simulink library "AtomicLibrary"
PostLoadFcn:
  | PacketBusGenerator; RailCabBusGenerator
(part 3 of 8)

== system AtomicLibrary/TestStartStopMaster/Link Layer startStop_Master ==
  port_in : Inport  Tag=id=_rqhdoPdmEeGH_6eRdlYQdA  Port=1  PortDimensions=-1  DataType=auto  OutDataType=fixdt(1, 16)  OutScaling=2^0  UseBusObject=on  OutDataTypeStr=Inherit: auto
      settings: BusObject=PacketBus
  net_address : Inport  Tag=id=_rqrOoPdmEeGH_6eRdlYQdA  Port=2  PortDimensions=-1  DataType=uint8  OutDataType=fixdt(1, 16)  OutScaling=2^0  OutDataTypeStr=uint8
  receiver_net_address : Inport  Tag=id=_rqr1sPdmEeGH_6eRdlYQdA  Port=3  PortDimensions=-1  DataType=uint8  OutDataType=fixdt(1, 16)  OutScaling=2^0  OutDataTypeStr=uint8
  read_event_queue_in : Inport  Tag=id=_rqiEsPdmEeGH_6eRdlYQdA  Port=4  PortDimensions=-1  DataType=auto  OutDataType=fixdt(1, 16)  OutScaling=2^0  OutDataTypeStr=Inherit: auto
  read_event_param_queue_in : Inport  Tag=id=_rqlvEPdmEeGH_6eRdlYQdA  Port=5  PortDimensions=-1  DataType=auto  OutDataType=fixdt(1, 16)  OutScaling=2^0  OutDataTypeStr=Inherit: auto
  read_event_queue_out : Inport  Tag=id=_rqnkQPdmEeGH_6eRdlYQdA  Port=6  PortDimensions=-1  DataType=auto  OutDataType=fixdt(1, 16)  OutScaling=2^0  OutDataTypeStr=Inherit: auto
  read_event_param_queue_out : Inport  Tag=id=_rqoyYPdmEeGH_6eRdlYQdA  Port=7  PortDimensions=-1  DataType=auto  OutDataType=fixdt(1, 16)  OutScaling=2^0  OutDataTypeStr=Inherit: auto
  port_out : Outport  Tag=id=_rqgPgPdmEeGH_6eRdlYQdA  Port=1  PortDimensions=-1  DataType=auto  OutDataType=fixdt(1, 16)  OutScaling=2^0  UseBusObject=on  OutDataTypeStr=Inherit: auto
      settings: BusObject=PacketBus
  write_event_queue_in : Outport  Tag=id=_rqjS0PdmEeGH_6eRdlYQdA  Port=2  PortDimensions=-1  DataType=auto  OutDataType=fixdt(1, 16)  OutScaling=2^0  OutDataTypeStr=Inherit: auto
  write_event_param_queue_in : Outport  Tag=id=_rqkg8PdmEeGH_6eRdlYQdA  Port=3  PortDimensions=-1  DataType=auto  OutDataType=fixdt(1, 16)  OutScaling=2^0  OutDataTypeStr=Inherit: auto
  write_event_queue_out : Outport  Tag=id=_rqpZcPdmEeGH_6eRdlYQdA  Port=4  PortDimensions=-1  DataType=auto  OutDataType=fixdt(1, 16)  OutScaling=2^0  OutDataTypeStr=Inherit: auto
  write_event_param_queue_out : Outport  Tag=id=_rqqAgPdmEeGH_6eRdlYQdA  Port=5  PortDimensions=-1  DataType=auto  OutDataType=fixdt(1, 16)  OutScaling=2^0  OutDataTypeStr=Inherit: auto
  DataLinkLayer : Subsystem  Tag=id=_rqtq4PdmEeGH_6eRdlYQdA
  Bus Selector : BusSelector  OutputSignals=from,to,msg,param,pkgid,time  Tag=id=_rqtD0PdmEeGH_6eRdlYQdA
  Unit Delay1 : UnitDelay  Tag=id=_rqtD0fdmEeGH_6eRdlYQdA  SampleTime=-1
  Unit Delay2 : UnitDelay  Tag=id=_rqtD0vdmEeGH_6eRdlYQdA  SampleTime=-1
  Unit Delay3 : UnitDelay  Tag=id=_rqtq4fdmEeGH_6eRdlYQdA  SampleTime=-1
  Bus Creator : BusCreator  Inputs=6  UseBusObject=on  Tag=id=_rquR8PdmEeGH_6eRdlYQdA
      settings: BusObject=PacketBus
  Unit Delay4 : UnitDelay  Tag=id=_rquR8fdmEeGH_6eRdlYQdA  SampleTime=-1
  Terminator : Terminator
      settings: Tag=id=_rquR8vdmEeGH_6eRdlYQdA
  Receive Packet : Stateflow chart  Tag=id=_rqu5APdmEeGH_6eRdlYQdA
  Send Packet : Stateflow chart  Tag=id=_rqu5AfdmEeGH_6eRdlYQdA
  wires:
  DataLinkLayer/3(snd_msg_out) -> Bus Creator/3
  DataLinkLayer/8(recv_msg_out) -> Receive Packet/2(packetMsg)
  Send Packet/3(eventQueue) -> Unit Delay1/1
  DataLinkLayer/7(recv_from_out) -> Receive Packet/1(packetFrom)
  Bus Selector/3 -> DataLinkLayer/3(recv_msg_in)
  read_event_param_queue_in/1 -> Receive Packet/5(eventParamQueueIn)
  Receive Packet/3(bufferOverflow) -> Terminator/1
  receiver_net_address/1 -> DataLinkLayer/8(snd_to_in)
  Receive Packet/2(eventParamQueue) -> Unit Delay4/1
  read_event_queue_out/1 -> Send Packet/2(eventQueueIn)
  DataLinkLayer/9(recv_param_out) -> Receive Packet/3(packetParam)
  Send Packet/2(packetParam) -> DataLinkLayer/10(snd_param_in)
  Bus Selector/2 -> DataLinkLayer/2(recv_to_in)
  port_in/1 -> Bus Selector/1
  read_event_param_queue_out/1 -> Send Packet/3(eventParamQueueIn)
  Send Packet/4(eventParamQueue) -> Unit Delay2/1
  Bus Selector/5 -> DataLinkLayer/5(recv_pkgid_in)
  Unit Delay4/1 -> write_event_param_queue_in/1
  read_event_queue_in/1 -> Receive Packet/4(eventQueueIn)
  Bus Selector/4 -> DataLinkLayer/4(recv_param_in)
  DataLinkLayer/2(snd_to_out) -> Bus Creator/2
  Bus Selector/6 -> DataLinkLayer/6(recv_time_in), Send Packet/1(busSizeSignal)
  Receive Packet/1(eventQueue) -> Unit Delay3/1
  DataLinkLayer/6(snd_time_out) -> Bus Creator/6
  Unit Delay1/1 -> write_event_queue_out/1
  DataLinkLayer/1(snd_from_out) -> Bus Creator/1
  DataLinkLayer/5(snd_pkgid_out) -> Bus Creator/5
  net_address/1 -> DataLinkLayer/7(snd_from_in)
  Send Packet/1(packetMsg) -> DataLinkLayer/9(snd_msg_in)
  Bus Creator/1 -> port_out/1  "Outport37"
  Unit Delay3/1 -> write_event_queue_in/1
  Bus Selector/1 -> DataLinkLayer/1(recv_from_in)
  Unit Delay2/1 -> write_event_param_queue_out/1
  DataLinkLayer/4(snd_param_out) -> Bus Creator/4

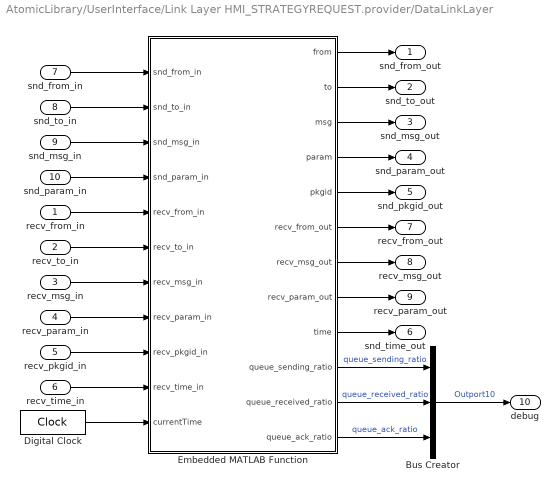
== system AtomicLibrary/UserInterface/Link Layer HMI_STRATEGYREQUEST.provider/DataLinkLayer ==
  recv_from_in : Inport  Tag=id=_r1VmgPdmEeGH_6eRdlYQdA  Port=1  PortDimensions=-1  DataType=uint8  OutDataType=fixdt(1, 16)  OutScaling=2^0  OutDataTypeStr=uint8
  recv_to_in : Inport  Tag=id=_r1XbsPdmEeGH_6eRdlYQdA  Port=2  PortDimensions=-1  DataType=uint8  OutDataType=fixdt(1, 16)  OutScaling=2^0  OutDataTypeStr=uint8
  recv_msg_in : Inport  Tag=id=_r1Yp0PdmEeGH_6eRdlYQdA  Port=3  PortDimensions=-1  DataType=uint16  OutDataType=fixdt(1, 16)  OutScaling=2^0  OutDataTypeStr=uint16
  recv_param_in : Inport  Tag=id=_r1afAPdmEeGH_6eRdlYQdA  Port=4  PortDimensions=-1  DataType=double  OutDataType=fixdt(1, 16)  OutScaling=2^0  OutDataTypeStr=double
  recv_pkgid_in : Inport  Tag=id=_r1cUMPdmEeGH_6eRdlYQdA  Port=5  PortDimensions=-1  DataType=uint32  OutDataType=fixdt(1, 16)  OutScaling=2^0  OutDataTypeStr=uint32
  recv_time_in : Inport  Tag=id=_r1eJYPdmEeGH_6eRdlYQdA  Port=6  PortDimensions=-1  DataType=double  OutDataType=fixdt(1, 16)  OutScaling=2^0  OutDataTypeStr=double
  snd_from_in : Inport  Tag=id=_r1f-kPdmEeGH_6eRdlYQdA  Port=7  PortDimensions=-1  DataType=uint8  OutDataType=fixdt(1, 16)  OutScaling=2^0  OutDataTypeStr=uint8
  snd_to_in : Inport  Tag=id=_r1hzwPdmEeGH_6eRdlYQdA  Port=8  PortDimensions=-1  DataType=uint8  OutDataType=fixdt(1, 16)  OutScaling=2^0  OutDataTypeStr=uint8
  snd_msg_in : Inport  Tag=id=_r1jo8PdmEeGH_6eRdlYQdA  Port=9  PortDimensions=-1  DataType=uint16  OutDataType=fixdt(1, 16)  OutScaling=2^0  OutDataTypeStr=uint16
  snd_param_in : Inport  Tag=id=_r1leIPdmEeGH_6eRdlYQdA  Port=10  PortDimensions=-1  DataType=double  OutDataType=fixdt(1, 16)  OutScaling=2^0  OutDataTypeStr=double
  snd_from_out : Outport  Tag=id=_r1LOcPdmEeGH_6eRdlYQdA  Port=1  PortDimensions=-1  DataType=uint8  OutDataType=fixdt(1, 16)  OutScaling=2^0  OutDataTypeStr=uint8
  snd_to_out : Outport  Tag=id=_r1L1gPdmEeGH_6eRdlYQdA  Port=2  PortDimensions=-1  DataType=uint8  OutDataType=fixdt(1, 16)  OutScaling=2^0  OutDataTypeStr=uint8
  snd_msg_out : Outport  Tag=id=_r1NDoPdmEeGH_6eRdlYQdA  Port=3  PortDimensions=-1  DataType=uint16  OutDataType=fixdt(1, 16)  OutScaling=2^0  OutDataTypeStr=uint16
  snd_param_out : Outport  Tag=id=_r1ORwPdmEeGH_6eRdlYQdA  Port=4  PortDimensions=-1  DataType=double  OutDataType=fixdt(1, 16)  OutScaling=2^0  OutDataTypeStr=double
  snd_pkgid_out : Outport  Tag=id=_r1Pf4PdmEeGH_6eRdlYQdA  Port=5  PortDimensions=-1  DataType=uint32  OutDataType=fixdt(1, 16)  OutScaling=2^0  OutDataTypeStr=uint32
  snd_time_out : Outport  Tag=id=_r1QG8PdmEeGH_6eRdlYQdA  Port=6  PortDimensions=-1  DataType=double  OutDataType=fixdt(1, 16)  OutScaling=2^0  OutDataTypeStr=double
  recv_from_out : Outport  Tag=id=_r1RVEPdmEeGH_6eRdlYQdA  Port=7  PortDimensions=-1  DataType=uint8  OutDataType=fixdt(1, 16)  OutScaling=2^0  OutDataTypeStr=uint8
  recv_msg_out : Outport  Tag=id=_r1SjMPdmEeGH_6eRdlYQdA  Port=8  PortDimensions=-1  DataType=uint16  OutDataType=fixdt(1, 16)  OutScaling=2^0  OutDataTypeStr=uint16
  recv_param_out : Outport  Tag=id=_r1TxUPdmEeGH_6eRdlYQdA  Port=9  PortDimensions=-1  DataType=double  OutDataType=fixdt(1, 16)  OutScaling=2^0  OutDataTypeStr=double
  debug : Outport  Tag=id=_r1UYYPdmEeGH_6eRdlYQdA  Port=10  PortDimensions=-1  DataType=auto  OutDataType=fixdt(1, 16)  OutScaling=2^0  OutDataTypeStr=Inherit: auto
  Bus Creator : BusCreator  Inputs=3  Tag=id=_r1msQPdmEeGH_6eRdlYQdA
  Embedded MATLAB Function : Stateflow chart  Tag=id=_r1msQfdmEeGH_6eRdlYQdA
  Digital Clock : DigitalClock  Tag=id=_r1pIgPdmEeGH_6eRdlYQdA  SampleTime=0.1
  wires:
  Embedded MATLAB Function/12(queue_ack_ratio) -> Bus Creator/3  "queue_ack_ratio"
  Embedded MATLAB Function/10(queue_sending_ratio) -> Bus Creator/1  "queue_sending_ratio"
  Embedded MATLAB Function/8(recv_param_out) -> recv_param_out/1
  recv_to_in/1 -> Embedded MATLAB Function/6(recv_to_in)
  Embedded MATLAB Function/5(pkgid) -> snd_pkgid_out/1
  snd_from_in/1 -> Embedded MATLAB Function/1(snd_from_in)
  Embedded MATLAB Function/7(recv_msg_out) -> recv_msg_out/1
  recv_pkgid_in/1 -> Embedded MATLAB Function/9(recv_pkgid_in)
  snd_msg_in/1 -> Embedded MATLAB Function/3(snd_msg_in)
  Digital Clock/1 -> Embedded MATLAB Function/11(currentTime)
  Embedded MATLAB Function/3(msg) -> snd_msg_out/1
  Embedded MATLAB Function/9(time) -> snd_time_out/1
  recv_from_in/1 -> Embedded MATLAB Function/5(recv_from_in)
  recv_time_in/1 -> Embedded MATLAB Function/10(recv_time_in)
  snd_to_in/1 -> Embedded MATLAB Function/2(snd_to_in)
  snd_param_in/1 -> Embedded MATLAB Function/4(snd_param_in)
  Embedded MATLAB Function/6(recv_from_out) -> recv_from_out/1
  recv_param_in/1 -> Embedded MATLAB Function/8(recv_param_in)
  Embedded MATLAB Function/2(to) -> snd_to_out/1
  recv_msg_in/1 -> Embedded MATLAB Function/7(recv_msg_in)
  Embedded MATLAB Function/4(param) -> snd_param_out/1
  Embedded MATLAB Function/1(from) -> snd_from_out/1
  Bus Creator/1 -> debug/1  "Outport10"
  Embedded MATLAB Function/11(queue_received_ratio) -> Bus Creator/2  "queue_received_ratio"

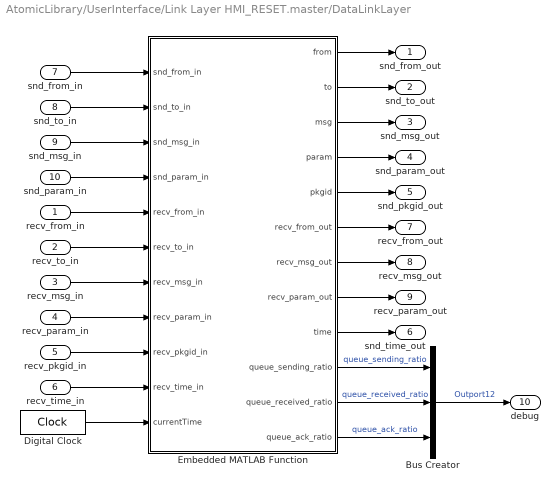
== system AtomicLibrary/UserInterface/Link Layer HMI_RESET.master/DataLinkLayer ==
  recv_from_in : Inport  Tag=id=_r_oK8PdmEeGH_6eRdlYQdA  Port=1  PortDimensions=-1  DataType=uint8  OutDataType=fixdt(1, 16)  OutScaling=2^0  OutDataTypeStr=uint8
  recv_to_in : Inport  Tag=id=_r_pZEPdmEeGH_6eRdlYQdA  Port=2  PortDimensions=-1  DataType=uint8  OutDataType=fixdt(1, 16)  OutScaling=2^0  OutDataTypeStr=uint8
  recv_msg_in : Inport  Tag=id=_r_qnMPdmEeGH_6eRdlYQdA  Port=3  PortDimensions=-1  DataType=uint16  OutDataType=fixdt(1, 16)  OutScaling=2^0  OutDataTypeStr=uint16
  recv_param_in : Inport  Tag=id=_r_scYPdmEeGH_6eRdlYQdA  Port=4  PortDimensions=-1  DataType=double  OutDataType=fixdt(1, 16)  OutScaling=2^0  OutDataTypeStr=double
  recv_pkgid_in : Inport  Tag=id=_r_tqgPdmEeGH_6eRdlYQdA  Port=5  PortDimensions=-1  DataType=uint32  OutDataType=fixdt(1, 16)  OutScaling=2^0  OutDataTypeStr=uint32
  recv_time_in : Inport  Tag=id=_r_vfsPdmEeGH_6eRdlYQdA  Port=6  PortDimensions=-1  DataType=double  OutDataType=fixdt(1, 16)  OutScaling=2^0  OutDataTypeStr=double
  snd_from_in : Inport  Tag=id=_r_wt0PdmEeGH_6eRdlYQdA  Port=7  PortDimensions=-1  DataType=uint8  OutDataType=fixdt(1, 16)  OutScaling=2^0  OutDataTypeStr=uint8
  snd_to_in : Inport  Tag=id=_r_yjAPdmEeGH_6eRdlYQdA  Port=8  PortDimensions=-1  DataType=uint8  OutDataType=fixdt(1, 16)  OutScaling=2^0  OutDataTypeStr=uint8
  snd_msg_in : Inport  Tag=id=_r_zxIPdmEeGH_6eRdlYQdA  Port=9  PortDimensions=-1  DataType=uint16  OutDataType=fixdt(1, 16)  OutScaling=2^0  OutDataTypeStr=uint16
  snd_param_in : Inport  Tag=id=_r_0_QPdmEeGH_6eRdlYQdA  Port=10  PortDimensions=-1  DataType=double  OutDataType=fixdt(1, 16)  OutScaling=2^0  OutDataTypeStr=double
  snd_from_out : Outport  Tag=id=_r_aIgPdmEeGH_6eRdlYQdA  Port=1  PortDimensions=-1  DataType=uint8  OutDataType=fixdt(1, 16)  OutScaling=2^0  OutDataTypeStr=uint8
  snd_to_out : Outport  Tag=id=_r_bWoPdmEeGH_6eRdlYQdA  Port=2  PortDimensions=-1  DataType=uint8  OutDataType=fixdt(1, 16)  OutScaling=2^0  OutDataTypeStr=uint8
  snd_msg_out : Outport  Tag=id=_r_b9sPdmEeGH_6eRdlYQdA  Port=3  PortDimensions=-1  DataType=uint16  OutDataType=fixdt(1, 16)  OutScaling=2^0  OutDataTypeStr=uint16
  snd_param_out : Outport  Tag=id=_r_dL0PdmEeGH_6eRdlYQdA  Port=4  PortDimensions=-1  DataType=double  OutDataType=fixdt(1, 16)  OutScaling=2^0  OutDataTypeStr=double
  snd_pkgid_out : Outport  Tag=id=_r_fBAPdmEeGH_6eRdlYQdA  Port=5  PortDimensions=-1  DataType=uint32  OutDataType=fixdt(1, 16)  OutScaling=2^0  OutDataTypeStr=uint32
  snd_time_out : Outport  Tag=id=_r_gPIPdmEeGH_6eRdlYQdA  Port=6  PortDimensions=-1  DataType=double  OutDataType=fixdt(1, 16)  OutScaling=2^0  OutDataTypeStr=double
  recv_from_out : Outport  Tag=id=_r_iEUPdmEeGH_6eRdlYQdA  Port=7  PortDimensions=-1  DataType=uint8  OutDataType=fixdt(1, 16)  OutScaling=2^0  OutDataTypeStr=uint8
  recv_msg_out : Outport  Tag=id=_r_jScPdmEeGH_6eRdlYQdA  Port=8  PortDimensions=-1  DataType=uint16  OutDataType=fixdt(1, 16)  OutScaling=2^0  OutDataTypeStr=uint16
  recv_param_out : Outport  Tag=id=_r_lHoPdmEeGH_6eRdlYQdA  Port=9  PortDimensions=-1  DataType=double  OutDataType=fixdt(1, 16)  OutScaling=2^0  OutDataTypeStr=double
  debug : Outport  Tag=id=_r_m80PdmEeGH_6eRdlYQdA  Port=10  PortDimensions=-1  DataType=auto  OutDataType=fixdt(1, 16)  OutScaling=2^0  OutDataTypeStr=Inherit: auto
  Bus Creator : BusCreator  Inputs=3  Tag=id=_r_3bgPdmEeGH_6eRdlYQdA
  Embedded MATLAB Function : Stateflow chart  Tag=id=_r_4CkPdmEeGH_6eRdlYQdA
  Digital Clock : DigitalClock  Tag=id=_r_7F4PdmEeGH_6eRdlYQdA  SampleTime=0.1
  wires:
  Embedded MATLAB Function/12(queue_ack_ratio) -> Bus Creator/3  "queue_ack_ratio"
  Embedded MATLAB Function/10(queue_sending_ratio) -> Bus Creator/1  "queue_sending_ratio"
  Embedded MATLAB Function/8(recv_param_out) -> recv_param_out/1
  recv_to_in/1 -> Embedded MATLAB Function/6(recv_to_in)
  Embedded MATLAB Function/5(pkgid) -> snd_pkgid_out/1
  snd_from_in/1 -> Embedded MATLAB Function/1(snd_from_in)
  Embedded MATLAB Function/7(recv_msg_out) -> recv_msg_out/1
  recv_pkgid_in/1 -> Embedded MATLAB Function/9(recv_pkgid_in)
  snd_msg_in/1 -> Embedded MATLAB Function/3(snd_msg_in)
  Digital Clock/1 -> Embedded MATLAB Function/11(currentTime)
  Embedded MATLAB Function/3(msg) -> snd_msg_out/1
  Embedded MATLAB Function/9(time) -> snd_time_out/1
  recv_from_in/1 -> Embedded MATLAB Function/5(recv_from_in)
  recv_time_in/1 -> Embedded MATLAB Function/10(recv_time_in)
  snd_to_in/1 -> Embedded MATLAB Function/2(snd_to_in)
  snd_param_in/1 -> Embedded MATLAB Function/4(snd_param_in)
  Embedded MATLAB Function/6(recv_from_out) -> recv_from_out/1
  recv_param_in/1 -> Embedded MATLAB Function/8(recv_param_in)
  Embedded MATLAB Function/2(to) -> snd_to_out/1
  recv_msg_in/1 -> Embedded MATLAB Function/7(recv_msg_in)
  Embedded MATLAB Function/4(param) -> snd_param_out/1
  Embedded MATLAB Function/1(from) -> snd_from_out/1
  Bus Creator/1 -> debug/1  "Outport12"
  Embedded MATLAB Function/11(queue_received_ratio) -> Bus Creator/2  "queue_received_ratio"

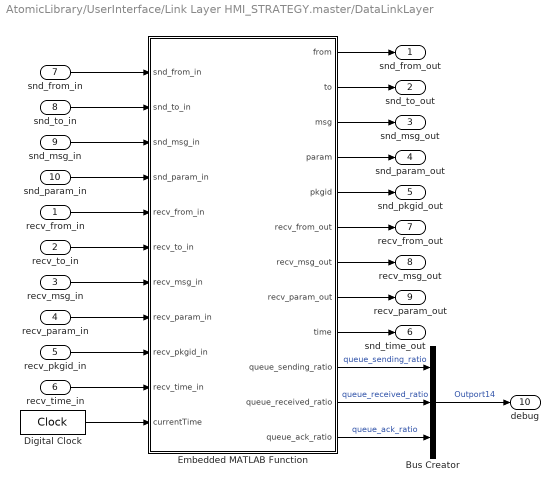
== system AtomicLibrary/UserInterface/Link Layer HMI_STRATEGY.master/DataLinkLayer ==
  recv_from_in : Inport  Tag=id=_sJ0owPdmEeGH_6eRdlYQdA  Port=1  PortDimensions=-1  DataType=uint8  OutDataType=fixdt(1, 16)  OutScaling=2^0  OutDataTypeStr=uint8
  recv_to_in : Inport  Tag=id=_sJ124PdmEeGH_6eRdlYQdA  Port=2  PortDimensions=-1  DataType=uint8  OutDataType=fixdt(1, 16)  OutScaling=2^0  OutDataTypeStr=uint8
  recv_msg_in : Inport  Tag=id=_sJ3FAPdmEeGH_6eRdlYQdA  Port=3  PortDimensions=-1  DataType=uint16  OutDataType=fixdt(1, 16)  OutScaling=2^0  OutDataTypeStr=uint16
  recv_param_in : Inport  Tag=id=_sJ4TIPdmEeGH_6eRdlYQdA  Port=4  PortDimensions=-1  DataType=double  OutDataType=fixdt(1, 16)  OutScaling=2^0  OutDataTypeStr=double
  recv_pkgid_in : Inport  Tag=id=_sJ5hQPdmEeGH_6eRdlYQdA  Port=5  PortDimensions=-1  DataType=uint32  OutDataType=fixdt(1, 16)  OutScaling=2^0  OutDataTypeStr=uint32
  recv_time_in : Inport  Tag=id=_sJ7WcPdmEeGH_6eRdlYQdA  Port=6  PortDimensions=-1  DataType=double  OutDataType=fixdt(1, 16)  OutScaling=2^0  OutDataTypeStr=double
  snd_from_in : Inport  Tag=id=_sJ9LoPdmEeGH_6eRdlYQdA  Port=7  PortDimensions=-1  DataType=uint8  OutDataType=fixdt(1, 16)  OutScaling=2^0  OutDataTypeStr=uint8
  snd_to_in : Inport  Tag=id=_sJ_A0PdmEeGH_6eRdlYQdA  Port=8  PortDimensions=-1  DataType=uint8  OutDataType=fixdt(1, 16)  OutScaling=2^0  OutDataTypeStr=uint8
  snd_msg_in : Inport  Tag=id=_sKA2APdmEeGH_6eRdlYQdA  Port=9  PortDimensions=-1  DataType=uint16  OutDataType=fixdt(1, 16)  OutScaling=2^0  OutDataTypeStr=uint16
  snd_param_in : Inport  Tag=id=_sKDSQPdmEeGH_6eRdlYQdA  Port=10  PortDimensions=-1  DataType=double  OutDataType=fixdt(1, 16)  OutScaling=2^0  OutDataTypeStr=double
  snd_from_out : Outport  Tag=id=_sJppoPdmEeGH_6eRdlYQdA  Port=1  PortDimensions=-1  DataType=uint8  OutDataType=fixdt(1, 16)  OutScaling=2^0  OutDataTypeStr=uint8
  snd_to_out : Outport  Tag=id=_sJq3wPdmEeGH_6eRdlYQdA  Port=2  PortDimensions=-1  DataType=uint8  OutDataType=fixdt(1, 16)  OutScaling=2^0  OutDataTypeStr=uint8
  snd_msg_out : Outport  Tag=id=_sJsF4PdmEeGH_6eRdlYQdA  Port=3  PortDimensions=-1  DataType=uint16  OutDataType=fixdt(1, 16)  OutScaling=2^0  OutDataTypeStr=uint16
  snd_param_out : Outport  Tag=id=_sJtUAPdmEeGH_6eRdlYQdA  Port=4  PortDimensions=-1  DataType=double  OutDataType=fixdt(1, 16)  OutScaling=2^0  OutDataTypeStr=double
  snd_pkgid_out : Outport  Tag=id=_sJt7EPdmEeGH_6eRdlYQdA  Port=5  PortDimensions=-1  DataType=uint32  OutDataType=fixdt(1, 16)  OutScaling=2^0  OutDataTypeStr=uint32
  snd_time_out : Outport  Tag=id=_sJvJMPdmEeGH_6eRdlYQdA  Port=6  PortDimensions=-1  DataType=double  OutDataType=fixdt(1, 16)  OutScaling=2^0  OutDataTypeStr=double
  recv_from_out : Outport  Tag=id=_sJwXUPdmEeGH_6eRdlYQdA  Port=7  PortDimensions=-1  DataType=uint8  OutDataType=fixdt(1, 16)  OutScaling=2^0  OutDataTypeStr=uint8
  recv_msg_out : Outport  Tag=id=_sJw-YPdmEeGH_6eRdlYQdA  Port=8  PortDimensions=-1  DataType=uint16  OutDataType=fixdt(1, 16)  OutScaling=2^0  OutDataTypeStr=uint16
  recv_param_out : Outport  Tag=id=_sJyMgPdmEeGH_6eRdlYQdA  Port=9  PortDimensions=-1  DataType=double  OutDataType=fixdt(1, 16)  OutScaling=2^0  OutDataTypeStr=double
  debug : Outport  Tag=id=_sJzaoPdmEeGH_6eRdlYQdA  Port=10  PortDimensions=-1  DataType=auto  OutDataType=fixdt(1, 16)  OutScaling=2^0  OutDataTypeStr=Inherit: auto
  Bus Creator : BusCreator  Inputs=3  Tag=id=_sKFHcPdmEeGH_6eRdlYQdA
  Embedded MATLAB Function : Stateflow chart  Tag=id=_sKFHcfdmEeGH_6eRdlYQdA
  Digital Clock : DigitalClock  Tag=id=_sKIx0PdmEeGH_6eRdlYQdA  SampleTime=0.1
  wires:
  Embedded MATLAB Function/12(queue_ack_ratio) -> Bus Creator/3  "queue_ack_ratio"
  Embedded MATLAB Function/10(queue_sending_ratio) -> Bus Creator/1  "queue_sending_ratio"
  Embedded MATLAB Function/8(recv_param_out) -> recv_param_out/1
  recv_to_in/1 -> Embedded MATLAB Function/6(recv_to_in)
  Embedded MATLAB Function/5(pkgid) -> snd_pkgid_out/1
  snd_from_in/1 -> Embedded MATLAB Function/1(snd_from_in)
  Embedded MATLAB Function/7(recv_msg_out) -> recv_msg_out/1
  recv_pkgid_in/1 -> Embedded MATLAB Function/9(recv_pkgid_in)
  snd_msg_in/1 -> Embedded MATLAB Function/3(snd_msg_in)
  Digital Clock/1 -> Embedded MATLAB Function/11(currentTime)
  Embedded MATLAB Function/3(msg) -> snd_msg_out/1
  Embedded MATLAB Function/9(time) -> snd_time_out/1
  recv_from_in/1 -> Embedded MATLAB Function/5(recv_from_in)
  recv_time_in/1 -> Embedded MATLAB Function/10(recv_time_in)
  snd_to_in/1 -> Embedded MATLAB Function/2(snd_to_in)
  snd_param_in/1 -> Embedded MATLAB Function/4(snd_param_in)
  Embedded MATLAB Function/6(recv_from_out) -> recv_from_out/1
  recv_param_in/1 -> Embedded MATLAB Function/8(recv_param_in)
  Embedded MATLAB Function/2(to) -> snd_to_out/1
  recv_msg_in/1 -> Embedded MATLAB Function/7(recv_msg_in)
  Embedded MATLAB Function/4(param) -> snd_param_out/1
  Embedded MATLAB Function/1(from) -> snd_from_out/1
  Bus Creator/1 -> debug/1  "Outport14"
  Embedded MATLAB Function/11(queue_received_ratio) -> Bus Creator/2  "queue_received_ratio"

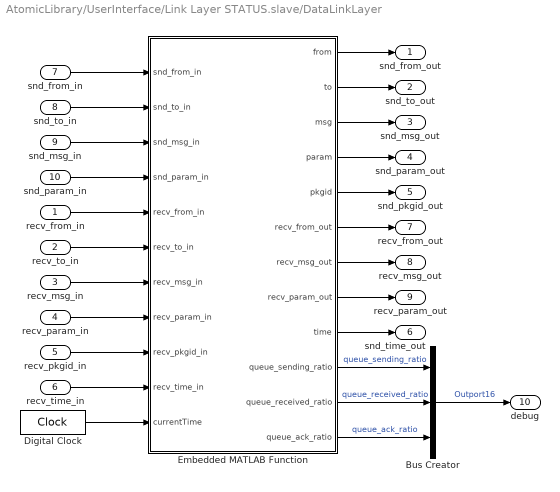
== system AtomicLibrary/UserInterface/Link Layer STATUS.slave/DataLinkLayer ==
  recv_from_in : Inport  Tag=id=_sUckYPdmEeGH_6eRdlYQdA  Port=1  PortDimensions=-1  DataType=uint8  OutDataType=fixdt(1, 16)  OutScaling=2^0  OutDataTypeStr=uint8
  recv_to_in : Inport  Tag=id=_sUdygPdmEeGH_6eRdlYQdA  Port=2  PortDimensions=-1  DataType=uint8  OutDataType=fixdt(1, 16)  OutScaling=2^0  OutDataTypeStr=uint8
  recv_msg_in : Inport  Tag=id=_sUfAoPdmEeGH_6eRdlYQdA  Port=3  PortDimensions=-1  DataType=uint16  OutDataType=fixdt(1, 16)  OutScaling=2^0  OutDataTypeStr=uint16
  recv_param_in : Inport  Tag=id=_sUgOwPdmEeGH_6eRdlYQdA  Port=4  PortDimensions=-1  DataType=double  OutDataType=fixdt(1, 16)  OutScaling=2^0  OutDataTypeStr=double
  recv_pkgid_in : Inport  Tag=id=_sUg10PdmEeGH_6eRdlYQdA  Port=5  PortDimensions=-1  DataType=uint32  OutDataType=fixdt(1, 16)  OutScaling=2^0  OutDataTypeStr=uint32
  recv_time_in : Inport  Tag=id=_sUiD8PdmEeGH_6eRdlYQdA  Port=6  PortDimensions=-1  DataType=double  OutDataType=fixdt(1, 16)  OutScaling=2^0  OutDataTypeStr=double
  snd_from_in : Inport  Tag=id=_sUjSEPdmEeGH_6eRdlYQdA  Port=7  PortDimensions=-1  DataType=uint8  OutDataType=fixdt(1, 16)  OutScaling=2^0  OutDataTypeStr=uint8
  snd_to_in : Inport  Tag=id=_sUkgMPdmEeGH_6eRdlYQdA  Port=8  PortDimensions=-1  DataType=uint8  OutDataType=fixdt(1, 16)  OutScaling=2^0  OutDataTypeStr=uint8
  snd_msg_in : Inport  Tag=id=_sUluUPdmEeGH_6eRdlYQdA  Port=9  PortDimensions=-1  DataType=uint16  OutDataType=fixdt(1, 16)  OutScaling=2^0  OutDataTypeStr=uint16
  snd_param_in : Inport  Tag=id=_sUm8cPdmEeGH_6eRdlYQdA  Port=10  PortDimensions=-1  DataType=double  OutDataType=fixdt(1, 16)  OutScaling=2^0  OutDataTypeStr=double
  snd_from_out : Outport  Tag=id=_sUPJAPdmEeGH_6eRdlYQdA  Port=1  PortDimensions=-1  DataType=uint8  OutDataType=fixdt(1, 16)  OutScaling=2^0  OutDataTypeStr=uint8
  snd_to_out : Outport  Tag=id=_sUQXIPdmEeGH_6eRdlYQdA  Port=2  PortDimensions=-1  DataType=uint8  OutDataType=fixdt(1, 16)  OutScaling=2^0  OutDataTypeStr=uint8
  snd_msg_out : Outport  Tag=id=_sUSMUPdmEeGH_6eRdlYQdA  Port=3  PortDimensions=-1  DataType=uint16  OutDataType=fixdt(1, 16)  OutScaling=2^0  OutDataTypeStr=uint16
  snd_param_out : Outport  Tag=id=_sUUBgPdmEeGH_6eRdlYQdA  Port=4  PortDimensions=-1  DataType=double  OutDataType=fixdt(1, 16)  OutScaling=2^0  OutDataTypeStr=double
  snd_pkgid_out : Outport  Tag=id=_sUVPoPdmEeGH_6eRdlYQdA  Port=5  PortDimensions=-1  DataType=uint32  OutDataType=fixdt(1, 16)  OutScaling=2^0  OutDataTypeStr=uint32
  snd_time_out : Outport  Tag=id=_sUXE0PdmEeGH_6eRdlYQdA  Port=6  PortDimensions=-1  DataType=double  OutDataType=fixdt(1, 16)  OutScaling=2^0  OutDataTypeStr=double
  recv_from_out : Outport  Tag=id=_sUYS8PdmEeGH_6eRdlYQdA  Port=7  PortDimensions=-1  DataType=uint8  OutDataType=fixdt(1, 16)  OutScaling=2^0  OutDataTypeStr=uint8
  recv_msg_out : Outport  Tag=id=_sUZhEPdmEeGH_6eRdlYQdA  Port=8  PortDimensions=-1  DataType=uint16  OutDataType=fixdt(1, 16)  OutScaling=2^0  OutDataTypeStr=uint16
  recv_param_out : Outport  Tag=id=_sUaIIPdmEeGH_6eRdlYQdA  Port=9  PortDimensions=-1  DataType=double  OutDataType=fixdt(1, 16)  OutScaling=2^0  OutDataTypeStr=double
  debug : Outport  Tag=id=_sUbWQPdmEeGH_6eRdlYQdA  Port=10  PortDimensions=-1  DataType=auto  OutDataType=fixdt(1, 16)  OutScaling=2^0  OutDataTypeStr=Inherit: auto
  Bus Creator : BusCreator  Inputs=3  Tag=id=_sUoKkPdmEeGH_6eRdlYQdA
  Embedded MATLAB Function : Stateflow chart  Tag=id=_sUoxoPdmEeGH_6eRdlYQdA
  Digital Clock : DigitalClock  Tag=id=_sUqm0PdmEeGH_6eRdlYQdA  SampleTime=0.1
  wires:
  Embedded MATLAB Function/12(queue_ack_ratio) -> Bus Creator/3  "queue_ack_ratio"
  Embedded MATLAB Function/10(queue_sending_ratio) -> Bus Creator/1  "queue_sending_ratio"
  Embedded MATLAB Function/8(recv_param_out) -> recv_param_out/1
  recv_to_in/1 -> Embedded MATLAB Function/6(recv_to_in)
  Embedded MATLAB Function/5(pkgid) -> snd_pkgid_out/1
  snd_from_in/1 -> Embedded MATLAB Function/1(snd_from_in)
  Embedded MATLAB Function/7(recv_msg_out) -> recv_msg_out/1
  recv_pkgid_in/1 -> Embedded MATLAB Function/9(recv_pkgid_in)
  snd_msg_in/1 -> Embedded MATLAB Function/3(snd_msg_in)
  Digital Clock/1 -> Embedded MATLAB Function/11(currentTime)
  Embedded MATLAB Function/3(msg) -> snd_msg_out/1
  Embedded MATLAB Function/9(time) -> snd_time_out/1
  recv_from_in/1 -> Embedded MATLAB Function/5(recv_from_in)
  recv_time_in/1 -> Embedded MATLAB Function/10(recv_time_in)
  snd_to_in/1 -> Embedded MATLAB Function/2(snd_to_in)
  snd_param_in/1 -> Embedded MATLAB Function/4(snd_param_in)
  Embedded MATLAB Function/6(recv_from_out) -> recv_from_out/1
  recv_param_in/1 -> Embedded MATLAB Function/8(recv_param_in)
  Embedded MATLAB Function/2(to) -> snd_to_out/1
  recv_msg_in/1 -> Embedded MATLAB Function/7(recv_msg_in)
  Embedded MATLAB Function/4(param) -> snd_param_out/1
  Embedded MATLAB Function/1(from) -> snd_from_out/1
  Bus Creator/1 -> debug/1  "Outport16"
  Embedded MATLAB Function/11(queue_received_ratio) -> Bus Creator/2  "queue_received_ratio"

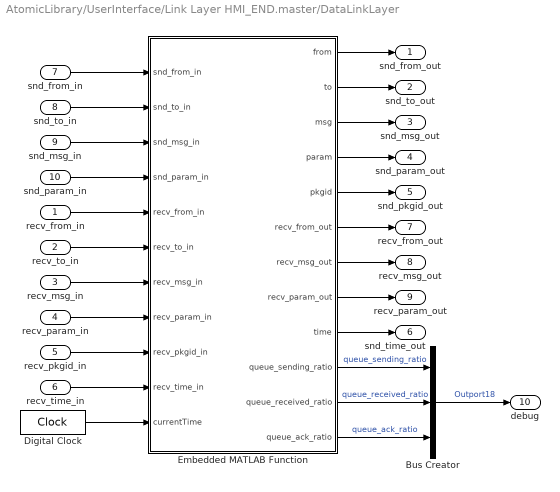
== system AtomicLibrary/UserInterface/Link Layer HMI_END.master/DataLinkLayer ==
  recv_from_in : Inport  Tag=id=_seQnsPdmEeGH_6eRdlYQdA  Port=1  PortDimensions=-1  DataType=uint8  OutDataType=fixdt(1, 16)  OutScaling=2^0  OutDataTypeStr=uint8
  recv_to_in : Inport  Tag=id=_seROwPdmEeGH_6eRdlYQdA  Port=2  PortDimensions=-1  DataType=uint8  OutDataType=fixdt(1, 16)  OutScaling=2^0  OutDataTypeStr=uint8
  recv_msg_in : Inport  Tag=id=_seTD8PdmEeGH_6eRdlYQdA  Port=3  PortDimensions=-1  DataType=uint16  OutDataType=fixdt(1, 16)  OutScaling=2^0  OutDataTypeStr=uint16
  recv_param_in : Inport  Tag=id=_seUSEPdmEeGH_6eRdlYQdA  Port=4  PortDimensions=-1  DataType=double  OutDataType=fixdt(1, 16)  OutScaling=2^0  OutDataTypeStr=double
  recv_pkgid_in : Inport  Tag=id=_seVgMPdmEeGH_6eRdlYQdA  Port=5  PortDimensions=-1  DataType=uint32  OutDataType=fixdt(1, 16)  OutScaling=2^0  OutDataTypeStr=uint32
  recv_time_in : Inport  Tag=id=_seWuUPdmEeGH_6eRdlYQdA  Port=6  PortDimensions=-1  DataType=double  OutDataType=fixdt(1, 16)  OutScaling=2^0  OutDataTypeStr=double
  snd_from_in : Inport  Tag=id=_seXVYPdmEeGH_6eRdlYQdA  Port=7  PortDimensions=-1  DataType=uint8  OutDataType=fixdt(1, 16)  OutScaling=2^0  OutDataTypeStr=uint8
  snd_to_in : Inport  Tag=id=_seYjgPdmEeGH_6eRdlYQdA  Port=8  PortDimensions=-1  DataType=uint8  OutDataType=fixdt(1, 16)  OutScaling=2^0  OutDataTypeStr=uint8
  snd_msg_in : Inport  Tag=id=_seaYsPdmEeGH_6eRdlYQdA  Port=9  PortDimensions=-1  DataType=uint16  OutDataType=fixdt(1, 16)  OutScaling=2^0  OutDataTypeStr=uint16
  snd_param_in : Inport  Tag=id=_secN4PdmEeGH_6eRdlYQdA  Port=10  PortDimensions=-1  DataType=double  OutDataType=fixdt(1, 16)  OutScaling=2^0  OutDataTypeStr=double
  snd_from_out : Outport  Tag=id=_seFokPdmEeGH_6eRdlYQdA  Port=1  PortDimensions=-1  DataType=uint8  OutDataType=fixdt(1, 16)  OutScaling=2^0  OutDataTypeStr=uint8
  snd_to_out : Outport  Tag=id=_seG2sPdmEeGH_6eRdlYQdA  Port=2  PortDimensions=-1  DataType=uint8  OutDataType=fixdt(1, 16)  OutScaling=2^0  OutDataTypeStr=uint8
  snd_msg_out : Outport  Tag=id=_seIE0PdmEeGH_6eRdlYQdA  Port=3  PortDimensions=-1  DataType=uint16  OutDataType=fixdt(1, 16)  OutScaling=2^0  OutDataTypeStr=uint16
  snd_param_out : Outport  Tag=id=_seIr4PdmEeGH_6eRdlYQdA  Port=4  PortDimensions=-1  DataType=double  OutDataType=fixdt(1, 16)  OutScaling=2^0  OutDataTypeStr=double
  snd_pkgid_out : Outport  Tag=id=_seJ6APdmEeGH_6eRdlYQdA  Port=5  PortDimensions=-1  DataType=uint32  OutDataType=fixdt(1, 16)  OutScaling=2^0  OutDataTypeStr=uint32
  snd_time_out : Outport  Tag=id=_seLIIPdmEeGH_6eRdlYQdA  Port=6  PortDimensions=-1  DataType=double  OutDataType=fixdt(1, 16)  OutScaling=2^0  OutDataTypeStr=double
  recv_from_out : Outport  Tag=id=_seLvMPdmEeGH_6eRdlYQdA  Port=7  PortDimensions=-1  DataType=uint8  OutDataType=fixdt(1, 16)  OutScaling=2^0  OutDataTypeStr=uint8
  recv_msg_out : Outport  Tag=id=_seM9UPdmEeGH_6eRdlYQdA  Port=8  PortDimensions=-1  DataType=uint16  OutDataType=fixdt(1, 16)  OutScaling=2^0  OutDataTypeStr=uint16
  recv_param_out : Outport  Tag=id=_seOLcPdmEeGH_6eRdlYQdA  Port=9  PortDimensions=-1  DataType=double  OutDataType=fixdt(1, 16)  OutScaling=2^0  OutDataTypeStr=double
  debug : Outport  Tag=id=_sePZkPdmEeGH_6eRdlYQdA  Port=10  PortDimensions=-1  DataType=auto  OutDataType=fixdt(1, 16)  OutScaling=2^0  OutDataTypeStr=Inherit: auto
  Bus Creator : BusCreator  Inputs=3  Tag=id=_seeDEPdmEeGH_6eRdlYQdA
  Embedded MATLAB Function : Stateflow chart  Tag=id=_seeqIPdmEeGH_6eRdlYQdA
  Digital Clock : DigitalClock  Tag=id=_seiUgPdmEeGH_6eRdlYQdA  SampleTime=0.1
  wires:
  Embedded MATLAB Function/12(queue_ack_ratio) -> Bus Creator/3  "queue_ack_ratio"
  Embedded MATLAB Function/10(queue_sending_ratio) -> Bus Creator/1  "queue_sending_ratio"
  Embedded MATLAB Function/8(recv_param_out) -> recv_param_out/1
  recv_to_in/1 -> Embedded MATLAB Function/6(recv_to_in)
  Embedded MATLAB Function/5(pkgid) -> snd_pkgid_out/1
  snd_from_in/1 -> Embedded MATLAB Function/1(snd_from_in)
  Embedded MATLAB Function/7(recv_msg_out) -> recv_msg_out/1
  recv_pkgid_in/1 -> Embedded MATLAB Function/9(recv_pkgid_in)
  snd_msg_in/1 -> Embedded MATLAB Function/3(snd_msg_in)
  Digital Clock/1 -> Embedded MATLAB Function/11(currentTime)
  Embedded MATLAB Function/3(msg) -> snd_msg_out/1
  Embedded MATLAB Function/9(time) -> snd_time_out/1
  recv_from_in/1 -> Embedded MATLAB Function/5(recv_from_in)
  recv_time_in/1 -> Embedded MATLAB Function/10(recv_time_in)
  snd_to_in/1 -> Embedded MATLAB Function/2(snd_to_in)
  snd_param_in/1 -> Embedded MATLAB Function/4(snd_param_in)
  Embedded MATLAB Function/6(recv_from_out) -> recv_from_out/1
  recv_param_in/1 -> Embedded MATLAB Function/8(recv_param_in)
  Embedded MATLAB Function/2(to) -> snd_to_out/1
  recv_msg_in/1 -> Embedded MATLAB Function/7(recv_msg_in)
  Embedded MATLAB Function/4(param) -> snd_param_out/1
  Embedded MATLAB Function/1(from) -> snd_from_out/1
  Bus Creator/1 -> debug/1  "Outport18"
  Embedded MATLAB Function/11(queue_received_ratio) -> Bus Creator/2  "queue_received_ratio"

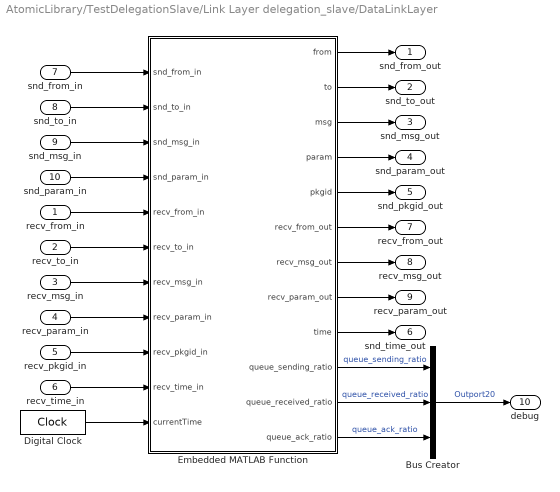
== system AtomicLibrary/TestDelegationSlave/Link Layer delegation_slave/DataLinkLayer ==
  recv_from_in : Inport  Tag=id=_qjYPYPdmEeGH_6eRdlYQdA  Port=1  PortDimensions=-1  DataType=uint8  OutDataType=fixdt(1, 16)  OutScaling=2^0  OutDataTypeStr=uint8
  recv_to_in : Inport  Tag=id=_qjaEkPdmEeGH_6eRdlYQdA  Port=2  PortDimensions=-1  DataType=uint8  OutDataType=fixdt(1, 16)  OutScaling=2^0  OutDataTypeStr=uint8
  recv_msg_in : Inport  Tag=id=_qjb5wPdmEeGH_6eRdlYQdA  Port=3  PortDimensions=-1  DataType=uint16  OutDataType=fixdt(1, 16)  OutScaling=2^0  OutDataTypeStr=uint16
  recv_param_in : Inport  Tag=id=_qjdH4PdmEeGH_6eRdlYQdA  Port=4  PortDimensions=-1  DataType=double  OutDataType=fixdt(1, 16)  OutScaling=2^0  OutDataTypeStr=double
  recv_pkgid_in : Inport  Tag=id=_qje9EPdmEeGH_6eRdlYQdA  Port=5  PortDimensions=-1  DataType=uint32  OutDataType=fixdt(1, 16)  OutScaling=2^0  OutDataTypeStr=uint32
  recv_time_in : Inport  Tag=id=_qjfkIPdmEeGH_6eRdlYQdA  Port=6  PortDimensions=-1  DataType=double  OutDataType=fixdt(1, 16)  OutScaling=2^0  OutDataTypeStr=double
  snd_from_in : Inport  Tag=id=_qjgyQPdmEeGH_6eRdlYQdA  Port=7  PortDimensions=-1  DataType=uint8  OutDataType=fixdt(1, 16)  OutScaling=2^0  OutDataTypeStr=uint8
  snd_to_in : Inport  Tag=id=_qjvbwPdmEeGH_6eRdlYQdA  Port=8  PortDimensions=-1  DataType=uint8  OutDataType=fixdt(1, 16)  OutScaling=2^0  OutDataTypeStr=uint8
  snd_msg_in : Inport  Tag=id=_qjwp4PdmEeGH_6eRdlYQdA  Port=9  PortDimensions=-1  DataType=uint16  OutDataType=fixdt(1, 16)  OutScaling=2^0  OutDataTypeStr=uint16
  snd_param_in : Inport  Tag=id=_qjx4APdmEeGH_6eRdlYQdA  Port=10  PortDimensions=-1  DataType=double  OutDataType=fixdt(1, 16)  OutScaling=2^0  OutDataTypeStr=double
  snd_from_out : Outport  Tag=id=_qjNQQPdmEeGH_6eRdlYQdA  Port=1  PortDimensions=-1  DataType=uint8  OutDataType=fixdt(1, 16)  OutScaling=2^0  OutDataTypeStr=uint8
  snd_to_out : Outport  Tag=id=_qjN3UPdmEeGH_6eRdlYQdA  Port=2  PortDimensions=-1  DataType=uint8  OutDataType=fixdt(1, 16)  OutScaling=2^0  OutDataTypeStr=uint8
  snd_msg_out : Outport  Tag=id=_qjPFcPdmEeGH_6eRdlYQdA  Port=3  PortDimensions=-1  DataType=uint16  OutDataType=fixdt(1, 16)  OutScaling=2^0  OutDataTypeStr=uint16
  snd_param_out : Outport  Tag=id=_qjPsgPdmEeGH_6eRdlYQdA  Port=4  PortDimensions=-1  DataType=double  OutDataType=fixdt(1, 16)  OutScaling=2^0  OutDataTypeStr=double
  snd_pkgid_out : Outport  Tag=id=_qjQ6oPdmEeGH_6eRdlYQdA  Port=5  PortDimensions=-1  DataType=uint32  OutDataType=fixdt(1, 16)  OutScaling=2^0  OutDataTypeStr=uint32
  snd_time_out : Outport  Tag=id=_qjSIwPdmEeGH_6eRdlYQdA  Port=6  PortDimensions=-1  DataType=double  OutDataType=fixdt(1, 16)  OutScaling=2^0  OutDataTypeStr=double
  recv_from_out : Outport  Tag=id=_qjSv0PdmEeGH_6eRdlYQdA  Port=7  PortDimensions=-1  DataType=uint8  OutDataType=fixdt(1, 16)  OutScaling=2^0  OutDataTypeStr=uint8
  recv_msg_out : Outport  Tag=id=_qjT98PdmEeGH_6eRdlYQdA  Port=8  PortDimensions=-1  DataType=uint16  OutDataType=fixdt(1, 16)  OutScaling=2^0  OutDataTypeStr=uint16
  recv_param_out : Outport  Tag=id=_qjVMEPdmEeGH_6eRdlYQdA  Port=9  PortDimensions=-1  DataType=double  OutDataType=fixdt(1, 16)  OutScaling=2^0  OutDataTypeStr=double
  debug : Outport  Tag=id=_qjXBQPdmEeGH_6eRdlYQdA  Port=10  PortDimensions=-1  DataType=auto  OutDataType=fixdt(1, 16)  OutScaling=2^0  OutDataTypeStr=Inherit: auto
  Bus Creator : BusCreator  Inputs=3  Tag=id=_qjztMPdmEeGH_6eRdlYQdA
  Embedded MATLAB Function : Stateflow chart  Tag=id=_qj0UQPdmEeGH_6eRdlYQdA
  Digital Clock : DigitalClock  Tag=id=_qj2wgPdmEeGH_6eRdlYQdA  SampleTime=0.1
  wires:
  Embedded MATLAB Function/12(queue_ack_ratio) -> Bus Creator/3  "queue_ack_ratio"
  Embedded MATLAB Function/10(queue_sending_ratio) -> Bus Creator/1  "queue_sending_ratio"
  Embedded MATLAB Function/8(recv_param_out) -> recv_param_out/1
  recv_to_in/1 -> Embedded MATLAB Function/6(recv_to_in)
  Embedded MATLAB Function/5(pkgid) -> snd_pkgid_out/1
  snd_from_in/1 -> Embedded MATLAB Function/1(snd_from_in)
  Embedded MATLAB Function/7(recv_msg_out) -> recv_msg_out/1
  recv_pkgid_in/1 -> Embedded MATLAB Function/9(recv_pkgid_in)
  snd_msg_in/1 -> Embedded MATLAB Function/3(snd_msg_in)
  Digital Clock/1 -> Embedded MATLAB Function/11(currentTime)
  Embedded MATLAB Function/3(msg) -> snd_msg_out/1
  Embedded MATLAB Function/9(time) -> snd_time_out/1
  recv_from_in/1 -> Embedded MATLAB Function/5(recv_from_in)
  recv_time_in/1 -> Embedded MATLAB Function/10(recv_time_in)
  snd_to_in/1 -> Embedded MATLAB Function/2(snd_to_in)
  snd_param_in/1 -> Embedded MATLAB Function/4(snd_param_in)
  Embedded MATLAB Function/6(recv_from_out) -> recv_from_out/1
  recv_param_in/1 -> Embedded MATLAB Function/8(recv_param_in)
  Embedded MATLAB Function/2(to) -> snd_to_out/1
  recv_msg_in/1 -> Embedded MATLAB Function/7(recv_msg_in)
  Embedded MATLAB Function/4(param) -> snd_param_out/1
  Embedded MATLAB Function/1(from) -> snd_from_out/1
  Bus Creator/1 -> debug/1  "Outport20"
  Embedded MATLAB Function/11(queue_received_ratio) -> Bus Creator/2  "queue_received_ratio"

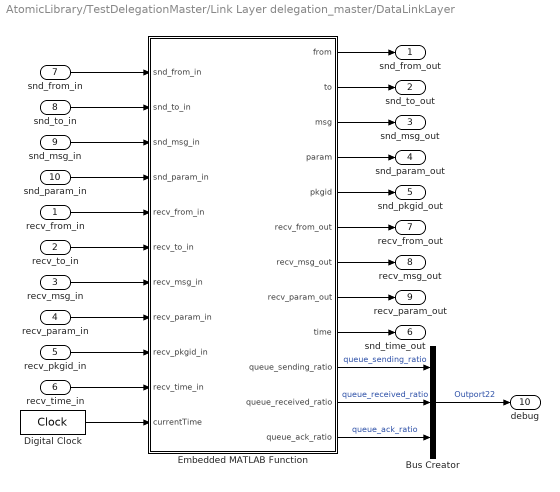
== system AtomicLibrary/TestDelegationMaster/Link Layer delegation_master/DataLinkLayer ==
  recv_from_in : Inport  Tag=id=_qsiLYPdmEeGH_6eRdlYQdA  Port=1  PortDimensions=-1  DataType=uint8  OutDataType=fixdt(1, 16)  OutScaling=2^0  OutDataTypeStr=uint8
  recv_to_in : Inport  Tag=id=_qsjZgPdmEeGH_6eRdlYQdA  Port=2  PortDimensions=-1  DataType=uint8  OutDataType=fixdt(1, 16)  OutScaling=2^0  OutDataTypeStr=uint8
  recv_msg_in : Inport  Tag=id=_qslOsPdmEeGH_6eRdlYQdA  Port=3  PortDimensions=-1  DataType=uint16  OutDataType=fixdt(1, 16)  OutScaling=2^0  OutDataTypeStr=uint16
  recv_param_in : Inport  Tag=id=_qsmc0PdmEeGH_6eRdlYQdA  Port=4  PortDimensions=-1  DataType=double  OutDataType=fixdt(1, 16)  OutScaling=2^0  OutDataTypeStr=double
  recv_pkgid_in : Inport  Tag=id=_qsoSAPdmEeGH_6eRdlYQdA  Port=5  PortDimensions=-1  DataType=uint32  OutDataType=fixdt(1, 16)  OutScaling=2^0  OutDataTypeStr=uint32
  recv_time_in : Inport  Tag=id=_qsqHMPdmEeGH_6eRdlYQdA  Port=6  PortDimensions=-1  DataType=double  OutDataType=fixdt(1, 16)  OutScaling=2^0  OutDataTypeStr=double
  snd_from_in : Inport  Tag=id=_qsrVUPdmEeGH_6eRdlYQdA  Port=7  PortDimensions=-1  DataType=uint8  OutDataType=fixdt(1, 16)  OutScaling=2^0  OutDataTypeStr=uint8
  snd_to_in : Inport  Tag=id=_qssjcPdmEeGH_6eRdlYQdA  Port=8  PortDimensions=-1  DataType=uint8  OutDataType=fixdt(1, 16)  OutScaling=2^0  OutDataTypeStr=uint8
  snd_msg_in : Inport  Tag=id=_qstxkPdmEeGH_6eRdlYQdA  Port=9  PortDimensions=-1  DataType=uint16  OutDataType=fixdt(1, 16)  OutScaling=2^0  OutDataTypeStr=uint16
  snd_param_in : Inport  Tag=id=_qsu_sPdmEeGH_6eRdlYQdA  Port=10  PortDimensions=-1  DataType=double  OutDataType=fixdt(1, 16)  OutScaling=2^0  OutDataTypeStr=double
  snd_from_out : Outport  Tag=id=_qsXMQPdmEeGH_6eRdlYQdA  Port=1  PortDimensions=-1  DataType=uint8  OutDataType=fixdt(1, 16)  OutScaling=2^0  OutDataTypeStr=uint8
  snd_to_out : Outport  Tag=id=_qsYaYPdmEeGH_6eRdlYQdA  Port=2  PortDimensions=-1  DataType=uint8  OutDataType=fixdt(1, 16)  OutScaling=2^0  OutDataTypeStr=uint8
  snd_msg_out : Outport  Tag=id=_qsZBcPdmEeGH_6eRdlYQdA  Port=3  PortDimensions=-1  DataType=uint16  OutDataType=fixdt(1, 16)  OutScaling=2^0  OutDataTypeStr=uint16
  snd_param_out : Outport  Tag=id=_qsZogPdmEeGH_6eRdlYQdA  Port=4  PortDimensions=-1  DataType=double  OutDataType=fixdt(1, 16)  OutScaling=2^0  OutDataTypeStr=double
  snd_pkgid_out : Outport  Tag=id=_qsa2oPdmEeGH_6eRdlYQdA  Port=5  PortDimensions=-1  DataType=uint32  OutDataType=fixdt(1, 16)  OutScaling=2^0  OutDataTypeStr=uint32
  snd_time_out : Outport  Tag=id=_qsbdsPdmEeGH_6eRdlYQdA  Port=6  PortDimensions=-1  DataType=double  OutDataType=fixdt(1, 16)  OutScaling=2^0  OutDataTypeStr=double
  recv_from_out : Outport  Tag=id=_qscr0PdmEeGH_6eRdlYQdA  Port=7  PortDimensions=-1  DataType=uint8  OutDataType=fixdt(1, 16)  OutScaling=2^0  OutDataTypeStr=uint8
  recv_msg_out : Outport  Tag=id=_qsd58PdmEeGH_6eRdlYQdA  Port=8  PortDimensions=-1  DataType=uint16  OutDataType=fixdt(1, 16)  OutScaling=2^0  OutDataTypeStr=uint16
  recv_param_out : Outport  Tag=id=_qsfIEPdmEeGH_6eRdlYQdA  Port=9  PortDimensions=-1  DataType=double  OutDataType=fixdt(1, 16)  OutScaling=2^0  OutDataTypeStr=double
  debug : Outport  Tag=id=_qsg9QPdmEeGH_6eRdlYQdA  Port=10  PortDimensions=-1  DataType=auto  OutDataType=fixdt(1, 16)  OutScaling=2^0  OutDataTypeStr=Inherit: auto
  Bus Creator : BusCreator  Inputs=3  Tag=id=_qsvmwPdmEeGH_6eRdlYQdA
  Embedded MATLAB Function : Stateflow chart  Tag=id=_qswN0PdmEeGH_6eRdlYQdA
  Digital Clock : DigitalClock  Tag=id=_qsyqEPdmEeGH_6eRdlYQdA  SampleTime=0.1
  wires:
  Embedded MATLAB Function/12(queue_ack_ratio) -> Bus Creator/3  "queue_ack_ratio"
  Embedded MATLAB Function/10(queue_sending_ratio) -> Bus Creator/1  "queue_sending_ratio"
  Embedded MATLAB Function/8(recv_param_out) -> recv_param_out/1
  recv_to_in/1 -> Embedded MATLAB Function/6(recv_to_in)
  Embedded MATLAB Function/5(pkgid) -> snd_pkgid_out/1
  snd_from_in/1 -> Embedded MATLAB Function/1(snd_from_in)
  Embedded MATLAB Function/7(recv_msg_out) -> recv_msg_out/1
  recv_pkgid_in/1 -> Embedded MATLAB Function/9(recv_pkgid_in)
  snd_msg_in/1 -> Embedded MATLAB Function/3(snd_msg_in)
  Digital Clock/1 -> Embedded MATLAB Function/11(currentTime)
  Embedded MATLAB Function/3(msg) -> snd_msg_out/1
  Embedded MATLAB Function/9(time) -> snd_time_out/1
  recv_from_in/1 -> Embedded MATLAB Function/5(recv_from_in)
  recv_time_in/1 -> Embedded MATLAB Function/10(recv_time_in)
  snd_to_in/1 -> Embedded MATLAB Function/2(snd_to_in)
  snd_param_in/1 -> Embedded MATLAB Function/4(snd_param_in)
  Embedded MATLAB Function/6(recv_from_out) -> recv_from_out/1
  recv_param_in/1 -> Embedded MATLAB Function/8(recv_param_in)
  Embedded MATLAB Function/2(to) -> snd_to_out/1
  recv_msg_in/1 -> Embedded MATLAB Function/7(recv_msg_in)
  Embedded MATLAB Function/4(param) -> snd_param_out/1
  Embedded MATLAB Function/1(from) -> snd_from_out/1
  Bus Creator/1 -> debug/1  "Outport22"
  Embedded MATLAB Function/11(queue_received_ratio) -> Bus Creator/2  "queue_received_ratio"

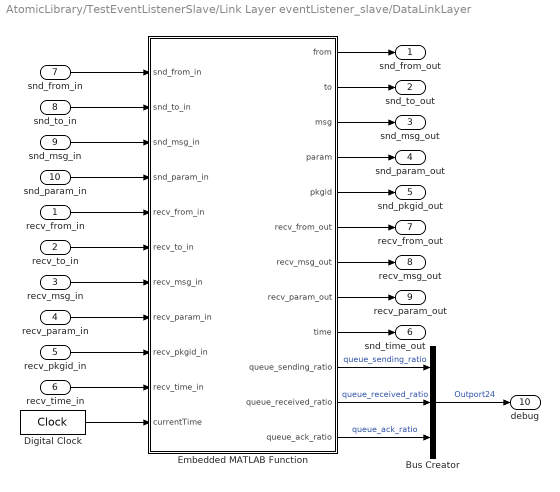
== system AtomicLibrary/TestEventListenerSlave/Link Layer eventListener_slave/DataLinkLayer ==
  recv_from_in : Inport  Tag=id=_q1lZsPdmEeGH_6eRdlYQdA  Port=1  PortDimensions=-1  DataType=uint8  OutDataType=fixdt(1, 16)  OutScaling=2^0  OutDataTypeStr=uint8
  recv_to_in : Inport  Tag=id=_q1nO4PdmEeGH_6eRdlYQdA  Port=2  PortDimensions=-1  DataType=uint8  OutDataType=fixdt(1, 16)  OutScaling=2^0  OutDataTypeStr=uint8
  recv_msg_in : Inport  Tag=id=_q1odAPdmEeGH_6eRdlYQdA  Port=3  PortDimensions=-1  DataType=uint16  OutDataType=fixdt(1, 16)  OutScaling=2^0  OutDataTypeStr=uint16
  recv_param_in : Inport  Tag=id=_q1qSMPdmEeGH_6eRdlYQdA  Port=4  PortDimensions=-1  DataType=double  OutDataType=fixdt(1, 16)  OutScaling=2^0  OutDataTypeStr=double
  recv_pkgid_in : Inport  Tag=id=_q1sHYPdmEeGH_6eRdlYQdA  Port=5  PortDimensions=-1  DataType=uint32  OutDataType=fixdt(1, 16)  OutScaling=2^0  OutDataTypeStr=uint32
  recv_time_in : Inport  Tag=id=_q1tVgPdmEeGH_6eRdlYQdA  Port=6  PortDimensions=-1  DataType=double  OutDataType=fixdt(1, 16)  OutScaling=2^0  OutDataTypeStr=double
  snd_from_in : Inport  Tag=id=_q1t8kPdmEeGH_6eRdlYQdA  Port=7  PortDimensions=-1  DataType=uint8  OutDataType=fixdt(1, 16)  OutScaling=2^0  OutDataTypeStr=uint8
  snd_to_in : Inport  Tag=id=_q1vKsPdmEeGH_6eRdlYQdA  Port=8  PortDimensions=-1  DataType=uint8  OutDataType=fixdt(1, 16)  OutScaling=2^0  OutDataTypeStr=uint8
  snd_msg_in : Inport  Tag=id=_q1wY0PdmEeGH_6eRdlYQdA  Port=9  PortDimensions=-1  DataType=uint16  OutDataType=fixdt(1, 16)  OutScaling=2^0  OutDataTypeStr=uint16
  snd_param_in : Inport  Tag=id=_q1w_4PdmEeGH_6eRdlYQdA  Port=10  PortDimensions=-1  DataType=double  OutDataType=fixdt(1, 16)  OutScaling=2^0  OutDataTypeStr=double
  snd_from_out : Outport  Tag=id=_q1XXQPdmEeGH_6eRdlYQdA  Port=1  PortDimensions=-1  DataType=uint8  OutDataType=fixdt(1, 16)  OutScaling=2^0  OutDataTypeStr=uint8
  snd_to_out : Outport  Tag=id=_q1YlYPdmEeGH_6eRdlYQdA  Port=2  PortDimensions=-1  DataType=uint8  OutDataType=fixdt(1, 16)  OutScaling=2^0  OutDataTypeStr=uint8
  snd_msg_out : Outport  Tag=id=_q1aakPdmEeGH_6eRdlYQdA  Port=3  PortDimensions=-1  DataType=uint16  OutDataType=fixdt(1, 16)  OutScaling=2^0  OutDataTypeStr=uint16
  snd_param_out : Outport  Tag=id=_q1bosPdmEeGH_6eRdlYQdA  Port=4  PortDimensions=-1  DataType=double  OutDataType=fixdt(1, 16)  OutScaling=2^0  OutDataTypeStr=double
  snd_pkgid_out : Outport  Tag=id=_q1c20PdmEeGH_6eRdlYQdA  Port=5  PortDimensions=-1  DataType=uint32  OutDataType=fixdt(1, 16)  OutScaling=2^0  OutDataTypeStr=uint32
  snd_time_out : Outport  Tag=id=_q1eE8PdmEeGH_6eRdlYQdA  Port=6  PortDimensions=-1  DataType=double  OutDataType=fixdt(1, 16)  OutScaling=2^0  OutDataTypeStr=double
  recv_from_out : Outport  Tag=id=_q1f6IPdmEeGH_6eRdlYQdA  Port=7  PortDimensions=-1  DataType=uint8  OutDataType=fixdt(1, 16)  OutScaling=2^0  OutDataTypeStr=uint8
  recv_msg_out : Outport  Tag=id=_q1hIQPdmEeGH_6eRdlYQdA  Port=8  PortDimensions=-1  DataType=uint16  OutDataType=fixdt(1, 16)  OutScaling=2^0  OutDataTypeStr=uint16
  recv_param_out : Outport  Tag=id=_q1iWYPdmEeGH_6eRdlYQdA  Port=9  PortDimensions=-1  DataType=double  OutDataType=fixdt(1, 16)  OutScaling=2^0  OutDataTypeStr=double
  debug : Outport  Tag=id=_q1kLkPdmEeGH_6eRdlYQdA  Port=10  PortDimensions=-1  DataType=auto  OutDataType=fixdt(1, 16)  OutScaling=2^0  OutDataTypeStr=Inherit: auto
  Bus Creator : BusCreator  Inputs=3  Tag=id=_q1yOAPdmEeGH_6eRdlYQdA
  Embedded MATLAB Function : Stateflow chart  Tag=id=_q1y1EPdmEeGH_6eRdlYQdA
  Digital Clock : DigitalClock  Tag=id=_q10qQPdmEeGH_6eRdlYQdA  SampleTime=0.1
  wires:
  Embedded MATLAB Function/12(queue_ack_ratio) -> Bus Creator/3  "queue_ack_ratio"
  Embedded MATLAB Function/10(queue_sending_ratio) -> Bus Creator/1  "queue_sending_ratio"
  Embedded MATLAB Function/8(recv_param_out) -> recv_param_out/1
  recv_to_in/1 -> Embedded MATLAB Function/6(recv_to_in)
  Embedded MATLAB Function/5(pkgid) -> snd_pkgid_out/1
  snd_from_in/1 -> Embedded MATLAB Function/1(snd_from_in)
  Embedded MATLAB Function/7(recv_msg_out) -> recv_msg_out/1
  recv_pkgid_in/1 -> Embedded MATLAB Function/9(recv_pkgid_in)
  snd_msg_in/1 -> Embedded MATLAB Function/3(snd_msg_in)
  Digital Clock/1 -> Embedded MATLAB Function/11(currentTime)
  Embedded MATLAB Function/3(msg) -> snd_msg_out/1
  Embedded MATLAB Function/9(time) -> snd_time_out/1
  recv_from_in/1 -> Embedded MATLAB Function/5(recv_from_in)
  recv_time_in/1 -> Embedded MATLAB Function/10(recv_time_in)
  snd_to_in/1 -> Embedded MATLAB Function/2(snd_to_in)
  snd_param_in/1 -> Embedded MATLAB Function/4(snd_param_in)
  Embedded MATLAB Function/6(recv_from_out) -> recv_from_out/1
  recv_param_in/1 -> Embedded MATLAB Function/8(recv_param_in)
  Embedded MATLAB Function/2(to) -> snd_to_out/1
  recv_msg_in/1 -> Embedded MATLAB Function/7(recv_msg_in)
  Embedded MATLAB Function/4(param) -> snd_param_out/1
  Embedded MATLAB Function/1(from) -> snd_from_out/1
  Bus Creator/1 -> debug/1  "Outport24"
  Embedded MATLAB Function/11(queue_received_ratio) -> Bus Creator/2  "queue_received_ratio"
